simulink model "Pendulum_SMC_18a"  (R2018a)
settings: Solver=VariableStepAuto  StartTime=0.0  StopTime=40  MaxStep=0.001  RelTol=1e-3
settings Model: Creator=Dell  LastModifiedBy=Dell
settings DataIOCC: ReturnWorkspaceOutputs=on
settings DebuggingCC: SFMachineParentedDataDiag=error
settings SFSimCC: SimUseLocalCustomCode=on
settings RTWCC: RTWUseLocalCustomCode=on

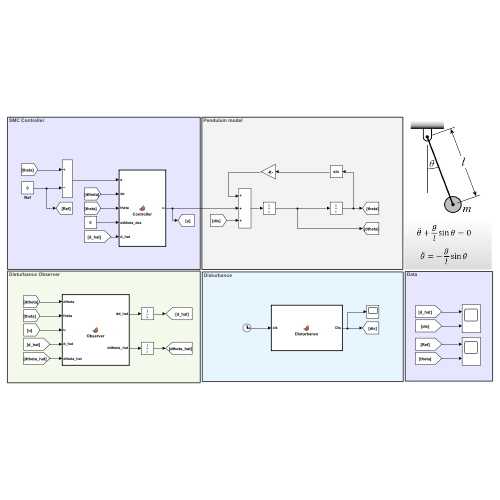
[thumbnail: Simulink's stored preview of the top-level diagram]
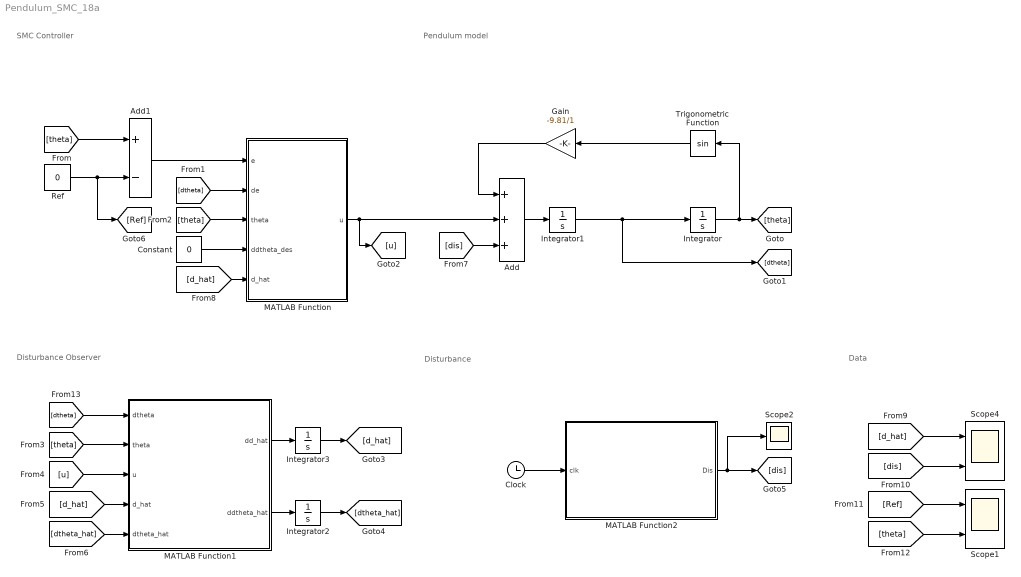
== system Pendulum_SMC_18a ==
  note: Data
  note: Disturbance
  note: Disturbance Observer
  note: Pendulum model
  note: SMC Controller
  Add : Sum  Inputs=+++
  Add1 : Sum  Inputs=+-
  Clock : Clock
  Constant : Constant  Value=0  SampleTime=-1
  Gain : Gain  Gain=-9.81/1
  Integrator : Integrator  InitialCondition=0.5
  Integrator1 : Integrator
  Integrator2 : Integrator  InitialCondition=0.5
  Integrator3 : Integrator
  MATLAB Function : MATLAB Function  TreatAsAtomicUnit=on
  MATLAB Function1 : MATLAB Function  TreatAsAtomicUnit=on
  MATLAB Function2 : MATLAB Function  TreatAsAtomicUnit=on
  Ref : Constant  Value=0  SampleTime=-1
  Scope1 : Scope  NumInputPorts=2
  Scope2 : Scope
  Scope4 : Scope  NumInputPorts=2
  Trigonometric Function : Trigonometry
  wires:
  Integrator/1 -> Trigonometric Function/1, [theta]
  Gain/1 -> Add/1
  Integrator1/1 -> Integrator/1, [dtheta]
  Trigonometric Function/1 -> Gain/1
  Add/1 -> Integrator1/1
  Ref/1 -> [Ref], Add1/2
  [theta] -> Add1/1
  Add1/1 -> MATLAB Function/1(e)
  [theta] -> MATLAB Function/3(theta)
  [dtheta] -> MATLAB Function1/1(dtheta)
  [u] -> MATLAB Function1/3(u)
  MATLAB Function1/2(ddtheta_hat) -> Integrator2/1
  MATLAB Function1/1(dd_hat) -> Integrator3/1
  Integrator3/1 -> [d_hat]
  [d_hat] -> MATLAB Function1/4(d_hat)
  Integrator2/1 -> [dtheta_hat]
  [dtheta_hat] -> MATLAB Function1/5(dtheta_hat)
  Clock/1 -> MATLAB Function2/1(clk)
  [dis] -> Add/3
  MATLAB Function2/1(Dis) -> Scope2/1, [dis]
  [d_hat] -> Scope4/1
  [dis] -> Scope4/2
  [Ref] -> Scope1/1
  [theta] -> Scope1/2
  [d_hat] -> MATLAB Function/5(d_hat)
  MATLAB Function/1(u) -> Add/2, [u]
  [theta] -> MATLAB Function1/2(theta)
  [dtheta] -> MATLAB Function/2(de)
  Constant/1 -> MATLAB Function/4(ddtheta_des)

== matlab function Pendulum_SMC_18a/MATLAB Function1 ==
  data: dtheta input; theta input; dd_hat output; ddtheta_hat output; u input; d_hat input; dtheta_hat input
function [dd_hat,ddtheta_hat] = Observer(dtheta,theta,u,d_hat,dtheta_hat)
%%%%%%%%%%%%%%%%%% params %%%%%%%%%%%%%%%%%%%%%
g=9.81;    l=1;
lambda1=3; lambda2=1; sigma1=0.01;
%%%%%%%%%%%%%%%%%%%%%%%%%%%%%%%%%%%%%%%%%%%%%%%

m=-lambda1*sqrt(abs(dtheta_hat-dtheta))*sign(dtheta_hat-dtheta)+d_hat;
dd_hat= -lambda2*sign(d_hat-m)-sigma1*d_hat;
ddtheta_hat=(-g/l)*sin(theta)+u+m;

== matlab function Pendulum_SMC_18a/MATLAB Function ==
  data: e input; u output; de input; theta input; ddtheta_des input; d_hat input
function u = Controller(e,de,theta, ddtheta_des, d_hat)

%%%%%%%%%%%%%%%%%%%%%%%%%%%%%%%% Params %%%%%%%%%%%%%%%%%%%%%%%%%%%%%%%%%%%%%% 
lambda=1;nu=0.4;g=9.81;l=1;epsilon=0.01;                                    
%%%%%%%%%%%%%%%%%%%%%%%%%%%%%%%%%%%%%%%%%%%%%%%%%%%%%%%%%%%%%%%%%%%%%%%%%%%%%%

S=de+lambda*e;
u =(g/l)*sin(theta)+ddtheta_des-lambda*de-nu*tanh(S/epsilon)-d_hat;


%%%%%%%%%%%%%%%%%%%%%%%%%%%%%%% remarks %%%%%%%%%%%%%%%%%%%%%%%%%%%%%%%%%%%%%%%
%  tanh(S/epsilon) is a smooth aproximation of sign() function                %
%                                                                             %
%  There is a tradeoff between Sign approximation and chattering phenomenon.  %
%  A smaller epsilon value leads to an improved approximation but introduces  %
%  more chattering in the control input.                                      %
%%%%%%%%%%%%%%%%%%%%%%%%%%%%%%%%%%%%%%%%%%%%%%%%%%%%%%%%%%%%%%%%%%%%%%%%%%%%%%%

== matlab function Pendulum_SMC_18a/MATLAB Function2 ==
  data: clk input; Dis output
function Dis = Disturbance(clk)

Dis = 0.2*sin(0.4*clk)+0.4*sin(clk);
